simulink model "esercizio3"  (Simulink 9.0)
settings: Solver=ode45  StartTime=0.0  StopTime=50  RelTol=1e-3  EnableMultiTasking=on
libraries: simulink x1
settings Model: Creator=DOC_CS31  LastModifiedBy=Matteo
settings DataIOCC: LimitDataPoints=on  SignalLoggingSaveFormat=ModelDataLogs
settings OptimizationCC: ExpressionDepthLimit=2147483647  InitFltsAndDblsToZero=on
settings DebuggingCC: SaveWithParameterizedLinksMsg=none  SolverPrmCheckMsg=warning  FcnCallInpInsideContextMsg=warning  StateNameClashWarn=warning
settings GRTTargetCC: TargetFcnLib=ansi_tfl_tmw.mat  GeneratePreprocessorConditionals=Disable all  CombineOutputUpdateFcns=off  GRTInterface=on

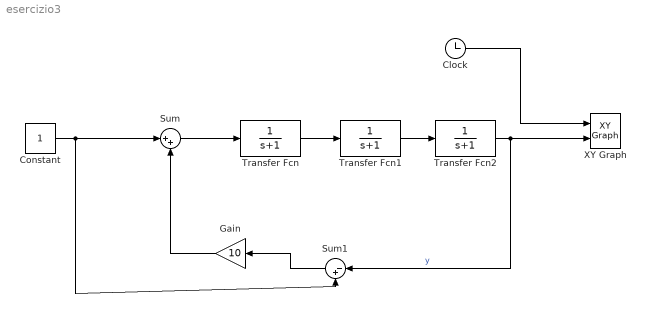
== system esercizio3 ==
  Clock : Clock
  Constant : Constant
  Gain : Gain  Gain=10
  Sum : Sum  Inputs=|++
  Sum1 : Sum  Inputs=|-+
  Transfer Fcn : TransferFcn  Denominator=[1 1]
  Transfer Fcn1 : TransferFcn  Denominator=[1 1]
  Transfer Fcn2 : TransferFcn  Denominator=[1 1]
  XY Graph : simulink/Sinks/XY Graph  xmin=0  xmax=50  ymin=-10  ymax=12  st=0.01
  wires:
  Constant/1 -> Sum/1, Sum1/2
  Transfer Fcn/1 -> Transfer Fcn1/1
  Transfer Fcn1/1 -> Transfer Fcn2/1
  Transfer Fcn2/1 -> Sum1/1, XY Graph/2  "y"
  Sum1/1 -> Gain/1
  Gain/1 -> Sum/2
  Clock/1 -> XY Graph/1
  Sum/1 -> Transfer Fcn/1
